simulink model "DUC_SIM"  (R2017b)
settings: Solver=VariableStepAuto  StartTime=0.0  StopTime=10.0  RelTol=1e-3
values from neighbouring files (symbols this model uses):
  A = 0.5*(nLev-1)    (= 0.5)    [Model3.m]
  ftest = 9e3    (= 9000)    [Model3.m]    (also in Model3_LTE.m = 2250)
undefined symbols (not defined in the file or in its folder): a, b, c, g
libraries: dspsigops x16, simulink x8, dspsrcs4 x1
(part 3 of 3)

== matlab function DUC_SIM/Delta_Sigma_Modulator1/Fourth_Order_Delta_Sigma_Modulator_Simulation/MATLAB Function ==
  data: u input; y output
function y = fcn(u)
%#codegen
% nLev=64;
% st=fi(nLev-2,1,36,28);
% y=fi(1,1,36,28);
% for n=1:nLev-2
%     k=fi(n,1,36,28);
%     if u < -st
%         y=fi(-nLev+1,1,36,28);
%         break;
%     elseif u > st
%         y=fi(nLev-1,1,36,28);
%         break;
%     elseif u >= -nLev + 2*k && u <= -nLev + 2*(k+1)
%         y=fi(2*k-1-nLev,1,36,28);
%         break;
%     end
% end

% 2-level
if u < 0
    y = fi(-1,1,36,32);
    %y = -1;
else
    y = fi(1,1,36,32);
    %y = 1;
end

% 4-level
% if u < -2
%     y = fi(-3,1,36,28);
% elseif u > -2 && u < 0
%     y = fi(-1,1,36,28);
% elseif u >= 0 && u < 2
%     y = fi(1,1,36,28);
% else
%     y = fi(3,1,36,28);
% end

% 64-level
% if u < -62
%     y = fi(-63,1,36,28);
% elseif u >= -62 && u < -60
%     y = fi(-61,1,36,28);
% elseif u >= -60 && u < -58
%     y = fi(-59,1,36,28);
% elseif u >= -58 && u < -56
%     y = fi(-57,1,36,28);
% elseif u >= -56 && u < -54
%     y = fi(-55,1,36,28);
% elseif u >= -54 && u < -52
%     y = fi(-53,1,36,28);
% elseif u >= -52 && u < -50
%     y = fi(-51,1,36,28);
% elseif u >= -50 && u < -48
%     y = fi(-49,1,36,28);
% elseif u >= -48 && u < -46
%     y = fi(-47,1,36,28);
% elseif u >= -46 && u < -44
%     y = fi(-45,1,36,28);
% elseif u >= -44 && u < -42
%     y = fi(-43,1,36,28);
% elseif u >= -42 && u < -40
%     y = fi(-41,1,36,28);
% elseif u >= -40 && u < -38
%     y = fi(-39,1,36,28);
% elseif u >= -38 && u < -36
%     y = fi(-37,1,36,28);
% elseif u >= -36 && u < -34
%     y = fi(-35,1,36,28);
% elseif u >= -34 && u < -32
%     y = fi(-33,1,36,28);
% elseif u >= -32 && u < -30
%     y = fi(-31,1,36,28);
% elseif u >= -30 && u < -28
%     y = fi(-29,1,36,28);
% elseif u >= -28 && u < -26
%     y = fi(-27,1,36,28);
% elseif u >= -26 && u < -24
%     y = fi(-25,1,36,28);
% elseif u >= -24 && u < -22
%     y = fi(-23,1,36,28);
% elseif u >= -22 && u < -20
%     y = fi(-21,1,36,28);
% elseif u >= -20 && u < -18
%     y = fi(-19,1,36,28);
% elseif u >= -18 && u < -16
%     y = fi(-17,1,36,28);
% elseif u >= -16 && u < -14
%     y = fi(-15,1,36,28);
% elseif u >= -14 && u < -12
%     y = fi(-13,1,36,28);
% elseif u >= -12 && u < -10
%     y = fi(-11,1,36,28);
% elseif u >= -10 && u < -8
%     y = fi(-9,1,36,28);
% elseif u >= -8 && u < -6
%     y = fi(-7,1,36,28);
% elseif u >= -6 && u < -4
%     y = fi(-5,1,36,28);
% elseif u >= -4 && u < -2
%     y = fi(-3,1,36,28);
% elseif u >= -2 && u < 0
%     y = fi(-1,1,36,28);
% elseif u >= 0 && u < 2
%     y = fi(1,1,36,28);
% elseif u >= 2 && u < 4
%     y = fi(3,1,36,28);
% elseif u >= 4 && u < 6
%     y = fi(5,1,36,28);
% elseif u >= 6 && u < 8
%     y = fi(7,1,36,28);
% elseif u >= 8 && u < 10
%     y = fi(9,1,36,28);
% elseif u >= 10 && u < 12
%     y = fi(11,1,36,28);
% elseif u >= 12 && u < 14
%     y = fi(13,1,36,28);
% elseif u >= 14 && u < 16
%     y = fi(15,1,36,28);
% elseif u >= 16 && u < 18
%     y = fi(17,1,36,28);
% elseif u >= 18 && u < 20
%     y = fi(19,1,36,28);
% elseif u >= 20 && u < 22
%     y = fi(21,1,36,28);
% elseif u >= 22 && u < 24
%     y = fi(23,1,36,28);
% elseif u >= 24 && u < 26
%     y = fi(25,1,36,28);
% elseif u >= 26 && u < 28
%     y = fi(27,1,36,28);
% elseif u >= 28 && u < 30
%     y = fi(29,1,36,28);
% elseif u >= 30 && u < 32
%     y = fi(31,1,36,28);
% elseif u >= 32 && u < 34
%     y = fi(33,1,36,28);
% elseif u >= 34 && u < 36
%     y = fi(35,1,36,28);
% elseif u >= 36 && u < 38
%     y = fi(37,1,36,28);
% elseif u >= 38 && u < 40
%     y = fi(39,1,36,28);
% elseif u >= 40 && u < 42
%     y = fi(41,1,36,28);
% elseif u >= 42 && u < 44
%     y = fi(43,1,36,28);
% elseif u >= 44 && u < 46
%     y = fi(45,1,36,28);
% elseif u >= 46 && u < 48
%     y = fi(47,1,36,28);
% elseif u >= 48 && u < 50
%     y = fi(49,1,36,28);
% elseif u >= 50 && u < 52
%     y = fi(51,1,36,28);
% elseif u >= 52 && u < 54
%     y = fi(53,1,36,28);
% elseif u >= 54 && u < 56
%     y = fi(55,1,36,28);
% elseif u >= 56 && u < 58
%     y = fi(57,1,36,28);
% elseif u >= 58 && u < 60
%     y = fi(59,1,36,28);
% elseif u >= 60 && u < 62
%     y = fi(61,1,36,28);
% else % u > 62
%     y = fi(63,1,36,28);
% end

% 32-level
% if u < -30
%     y = fi(-31,1,36,28);
% elseif u >= -30 && u < -28
%     y = fi(-29,1,36,28);
% elseif u >= -28 && u < -26
%     y = fi(-27,1,36,28);
% elseif u >= -26 && u < -24
%     y = fi(-25,1,36,28);
% elseif u >= -24 && u < -22
%     y = fi(-23,1,36,28);
% elseif u >= -22 && u < -20
%     y = fi(-21,1,36,28);
% elseif u >= -20 && u < -18
%     y = fi(-19,1,36,28);
% elseif u >= -18 && u < -16
%     y = fi(-17,1,36,28);
% elseif u >= -16 && u < -14
%     y = fi(-15,1,36,28);
% elseif u >= -14 && u < -12
%     y = fi(-13,1,36,28);
% elseif u >= -12 && u < -10
%     y = fi(-11,1,36,28);
% elseif u >= -10 && u < -8
%     y = fi(-9,1,36,28);
% elseif u >= -8 && u < -6
%     y = fi(-7,1,36,28);
% elseif u >= -6 && u < -4
%     y = fi(-5,1,36,28);
% elseif u >= -4 && u < -2
%     y = fi(-3,1,36,28);
% elseif u >= -2 && u < 0
%     y = fi(-1,1,36,28);
% elseif u >= 0 && u < 2
%     y = fi(1,1,36,28);
% elseif u >= 2 && u < 4
%     y = fi(3,1,36,28);
% elseif u >= 4 && u < 6
%     y = fi(5,1,36,28);
% elseif u >= 6 && u < 8
%     y = fi(7,1,36,28);
% elseif u >= 8 && u < 10
%     y = fi(9,1,36,28);
% elseif u >= 10 && u < 12
%     y = fi(11,1,36,28);
% elseif u >= 12 && u < 14
%     y = fi(13,1,36,28);
% elseif u >= 14 && u < 16
%     y = fi(15,1,36,28);
% elseif u >= 16 && u < 18
%     y = fi(17,1,36,28);
% elseif u >= 18 && u < 20
%     y = fi(19,1,36,28);
% elseif u >= 20 && u < 22
%     y = fi(21,1,36,28);
% elseif u >= 22 && u < 24
%     y = fi(23,1,36,28);
% elseif u >= 24 && u < 26
%     y = fi(25,1,36,28);
% elseif u >= 26 && u < 28
%     y = fi(27,1,36,28);
% elseif u >= 28 && u < 30
%     y = fi(29,1,36,28);
% else % u > 30
%     y = fi(31,1,36,28);
% end

== matlab function DUC_SIM/Delta_Sigma_Modulator1/Second_Order_Delta_Sigma_Modulator_Simulation/MATLAB Function ==
  data: u input; y output
function y = fcn(u)
%#codegen
% nLev=2;
% st=fi(nLev-2,1,36,30);
% y=fi(0,1,36,30);
% if u < -st
%     y = fi(-nLev+1,1,36,30);
% elseif u >= st
%     y = fi(nLev-1,1,36,30);
% else
%     for n=1:nLev-2
%         k=fi(n,1,36,30);
%         if u >= -nLev + 2*k && u < -nLev + 2*(k+1)
%             y = fi(2*k-1-nLev,1,36,30);
%         end
%     end
% end
% nLev=64;
% st=fi(nLev-2,1,36,25);
% y=fi(0,1,36,25);
% for n=1:nLev-2
%     k=fi(n,1,36,25);
%     if u < -st
%         y = fi(-nLev+1,1,36,25);
%         break;
%     elseif u >= st
%         y = fi(nLev-1,1,36,25);
%         break;
%     elseif u >= -nLev + 2*k && u < -nLev + 2*(k+1)
%         y = fi(2*k-1-nLev,1,36,25);
%         break;
%     end
% end

if u < 0
    y = fi(-1,1,36,32);
    %y = -1;
else
    y = fi(1,1,36,32);
    %y = 1;
end

% if u < -14
%     y = fi(-15,1,36,28);
% elseif u >= -14 && u < -12
%     y = fi(-13,1,36,28);
% elseif u >= -12 && u < -10
%     y = fi(-11,1,36,28);
% elseif u >= -10 && u < -8
%     y = fi(-9,1,36,28);
% elseif u >= -8 && u < -6
%     y = fi(-7,1,36,28);
% elseif u >= -6 && u < -4
%     y = fi(-5,1,36,28);
% elseif u >= -4 && u < -2
%     y = fi(-3,1,36,28);
% elseif u >= -2 && u < 0
%     y = fi(-1,1,36,28);
% elseif u >= 0 && u < 2
%     y = fi(1,1,36,28);
% elseif u >= 2 && u < 4
%     y = fi(3,1,36,28);
% elseif u >= 4 && u < 6
%     y = fi(5,1,36,28);
% elseif u >= 6 && u < 8
%     y = fi(7,1,36,28);
% elseif u >= 8 && u < 10
%     y = fi(9,1,36,28);
% elseif u >= 10 && u < 12
%     y = fi(11,1,36,28);
% elseif u >= 12 && u < 14
%     y = fi(13,1,36,28);
% else % u > 14
%     y = fi(15,1,36,28);
% end

== matlab function DUC_SIM/Delta_Sigma_Modulator2/Eight_Order_Delta_Sigma_Modulator/MATLAB Function ==
  data: u input; y output
function y = fcn(u)
%#codegen
% nLev=32;
% st=fi(nLev-2,1,36,28);
% y=fi(1,1,36,28);
% for n=1:nLev-2
%     k=fi(n,1,36,28);
%     if u < -st
%         y=fi(-nLev+1,1,36,28);
%         break;
%     elseif u > st
%         y=fi(nLev-1,1,36,28);
%         break;
%     elseif u >= -nLev + 2*k && u <= -nLev + 2*(k+1)
%         y=fi(2*k-1-nLev,1,36,28);
%         break;
%     end
% end
% nLev=2;
% st=fi(nLev,1,36,28);
% y=fi(0,1,36,28);
% for n=1:nLev
%     k=fi(n,1,36,28);
%     if u < -st+2
%         y = fi(-nLev+1,1,36,28);
%         break;
%     elseif u < -nLev + 2*k && u > -nLev + 2*(k+1)
%         y = fi(-nLev+1,1,36,28);
%         break;
%     elseif u >= nLev - 2*k && u < nLev - 2*(k+1)
%         y = fi(-nLev+1,1,36,28);
%         break;
%     else u > st-2
%         y = fi(nLev-1,1,36,28);
%         break;
%     end
% end

% 2-level
% if u < 0
%     y = -1;
% else
%     y = 1;
% end

% 2-level
if u < 0
    y = fi(-1,1,36,32);
else
    y = fi(1,1,36,32);
end

% 4-level
% if u < -2
%     y = fi(-3,1,36,28);
% elseif u > -2 && u < 0
%     y = fi(-1,1,36,28);
% elseif u >= 0 && u < 2
%     y = fi(1,1,36,28);
% else
%     y = fi(3,1,36,28);
% end

% 64-level
% if u < -62
%     y = fi(-63,1,36,28);
% elseif u >= -62 && u < -60
%     y = fi(-61,1,36,28);
% elseif u >= -60 && u < -58
%     y = fi(-59,1,36,28);
% elseif u >= -58 && u < -56
%     y = fi(-57,1,36,28);
% elseif u >= -56 && u < -54
%     y = fi(-55,1,36,28);
% elseif u >= -54 && u < -52
%     y = fi(-53,1,36,28);
% elseif u >= -52 && u < -50
%     y = fi(-51,1,36,28);
% elseif u >= -50 && u < -48
%     y = fi(-49,1,36,28);
% elseif u >= -48 && u < -46
%     y = fi(-47,1,36,28);
% elseif u >= -46 && u < -44
%     y = fi(-45,1,36,28);
% elseif u >= -44 && u < -42
%     y = fi(-43,1,36,28);
% elseif u >= -42 && u < -40
%     y = fi(-41,1,36,28);
% elseif u >= -40 && u < -38
%     y = fi(-39,1,36,28);
% elseif u >= -38 && u < -36
%     y = fi(-37,1,36,28);
% elseif u >= -36 && u < -34
%     y = fi(-35,1,36,28);
% elseif u >= -34 && u < -32
%     y = fi(-33,1,36,28);
% elseif u >= -32 && u < -30
%     y = fi(-31,1,36,28);
% elseif u >= -30 && u < -28
%     y = fi(-29,1,36,28);
% elseif u >= -28 && u < -26
%     y = fi(-27,1,36,28);
% elseif u >= -26 && u < -24
%     y = fi(-25,1,36,28);
% elseif u >= -24 && u < -22
%     y = fi(-23,1,36,28);
% elseif u >= -22 && u < -20
%     y = fi(-21,1,36,28);
% elseif u >= -20 && u < -18
%     y = fi(-19,1,36,28);
% elseif u >= -18 && u < -16
%     y = fi(-17,1,36,28);
% elseif u >= -16 && u < -14
%     y = fi(-15,1,36,28);
% elseif u >= -14 && u < -12
%     y = fi(-13,1,36,28);
% elseif u >= -12 && u < -10
%     y = fi(-11,1,36,28);
% elseif u >= -10 && u < -8
%     y = fi(-9,1,36,28);
% elseif u >= -8 && u < -6
%     y = fi(-7,1,36,28);
% elseif u >= -6 && u < -4
%     y = fi(-5,1,36,28);
% elseif u >= -4 && u < -2
%     y = fi(-3,1,36,28);
% elseif u >= -2 && u < 0
%     y = fi(-1,1,36,28);
% elseif u >= 0 && u < 2
%     y = fi(1,1,36,28);
% elseif u >= 2 && u < 4
%     y = fi(3,1,36,28);
% elseif u >= 4 && u < 6
%     y = fi(5,1,36,28);
% elseif u >= 6 && u < 8
%     y = fi(7,1,36,28);
% elseif u >= 8 && u < 10
%     y = fi(9,1,36,28);
% elseif u >= 10 && u < 12
%     y = fi(11,1,36,28);
% elseif u >= 12 && u < 14
%     y = fi(13,1,36,28);
% elseif u >= 14 && u < 16
%     y = fi(15,1,36,28);
% elseif u >= 16 && u < 18
%     y = fi(17,1,36,28);
% elseif u >= 18 && u < 20
%     y = fi(19,1,36,28);
% elseif u >= 20 && u < 22
%     y = fi(21,1,36,28);
% elseif u >= 22 && u < 24
%     y = fi(23,1,36,28);
% elseif u >= 24 && u < 26
%     y = fi(25,1,36,28);
% elseif u >= 26 && u < 28
%     y = fi(27,1,36,28);
% elseif u >= 28 && u < 30
%     y = fi(29,1,36,28);
% elseif u >= 30 && u < 32
%     y = fi(31,1,36,28);
% elseif u >= 32 && u < 34
%     y = fi(33,1,36,28);
% elseif u >= 34 && u < 36
%     y = fi(35,1,36,28);
% elseif u >= 36 && u < 38
%     y = fi(37,1,36,28);
% elseif u >= 38 && u < 40
%     y = fi(39,1,36,28);
% elseif u >= 40 && u < 42
%     y = fi(41,1,36,28);
% elseif u >= 42 && u < 44
%     y = fi(43,1,36,28);
% elseif u >= 44 && u < 46
%     y = fi(45,1,36,28);
% elseif u >= 46 && u < 48
%     y = fi(47,1,36,28);
% elseif u >= 48 && u < 50
%     y = fi(49,1,36,28);
% elseif u >= 50 && u < 52
%     y = fi(51,1,36,28);
% elseif u >= 52 && u < 54
%     y = fi(53,1,36,28);
% elseif u >= 54 && u < 56
%     y = fi(55,1,36,28);
% elseif u >= 56 && u < 58
%     y = fi(57,1,36,28);
% elseif u >= 58 && u < 60
%     y = fi(59,1,36,28);
% elseif u >= 60 && u < 62
%     y = fi(61,1,36,28);
% else % u > 62
%     y = fi(63,1,36,28);
% end

% 32-level
% if u < -30
%     y = fi(-31,1,36,28);
% elseif u >= -30 && u < -28
%     y = fi(-29,1,36,28);
% elseif u >= -28 && u < -26
%     y = fi(-27,1,36,28);
% elseif u >= -26 && u < -24
%     y = fi(-25,1,36,28);
% elseif u >= -24 && u < -22
%     y = fi(-23,1,36,28);
% elseif u >= -22 && u < -20
%     y = fi(-21,1,36,28);
% elseif u >= -20 && u < -18
%     y = fi(-19,1,36,28);
% elseif u >= -18 && u < -16
%     y = fi(-17,1,36,28);
% elseif u >= -16 && u < -14
%     y = fi(-15,1,36,28);
% elseif u >= -14 && u < -12
%     y = fi(-13,1,36,28);
% elseif u >= -12 && u < -10
%     y = fi(-11,1,36,28);
% elseif u >= -10 && u < -8
%     y = fi(-9,1,36,28);
% elseif u >= -8 && u < -6
%     y = fi(-7,1,36,28);
% elseif u >= -6 && u < -4
%     y = fi(-5,1,36,28);
% elseif u >= -4 && u < -2
%     y = fi(-3,1,36,28);
% elseif u >= -2 && u < 0
%     y = fi(-1,1,36,28);
% elseif u >= 0 && u < 2
%     y = fi(1,1,36,28);
% elseif u >= 2 && u < 4
%     y = fi(3,1,36,28);
% elseif u >= 4 && u < 6
%     y = fi(5,1,36,28);
% elseif u >= 6 && u < 8
%     y = fi(7,1,36,28);
% elseif u >= 8 && u < 10
%     y = fi(9,1,36,28);
% elseif u >= 10 && u < 12
%     y = fi(11,1,36,28);
% elseif u >= 12 && u < 14
%     y = fi(13,1,36,28);
% elseif u >= 14 && u < 16
%     y = fi(15,1,36,28);
% elseif u >= 16 && u < 18
%     y = fi(17,1,36,28);
% elseif u >= 18 && u < 20
%     y = fi(19,1,36,28);
% elseif u >= 20 && u < 22
%     y = fi(21,1,36,28);
% elseif u >= 22 && u < 24
%     y = fi(23,1,36,28);
% elseif u >= 24 && u < 26
%     y = fi(25,1,36,28);
% elseif u >= 26 && u < 28
%     y = fi(27,1,36,28);
% elseif u >= 28 && u < 30
%     y = fi(29,1,36,28);
% else % u > 30
%     y = fi(31,1,36,28);
% end

== matlab function DUC_SIM/Delta_Sigma_Modulator2/Fourth_Order_Delta_Sigma_Modulator_Simulation/MATLAB Function ==
  data: u input; y output
function y = fcn(u)
%#codegen
% nLev=64;
% st=fi(nLev-2,1,36,28);
% y=fi(1,1,36,28);
% for n=1:nLev-2
%     k=fi(n,1,36,28);
%     if u < -st
%         y=fi(-nLev+1,1,36,28);
%         break;
%     elseif u > st
%         y=fi(nLev-1,1,36,28);
%         break;
%     elseif u >= -nLev + 2*k && u <= -nLev + 2*(k+1)
%         y=fi(2*k-1-nLev,1,36,28);
%         break;
%     end
% end

% 2-level
if u < 0
    y = fi(-1,1,36,32);
    %y = -1;
else
    y = fi(1,1,36,32);
    %y = 1;
end

% 4-level
% if u < -2
%     y = fi(-3,1,36,28);
% elseif u > -2 && u < 0
%     y = fi(-1,1,36,28);
% elseif u >= 0 && u < 2
%     y = fi(1,1,36,28);
% else
%     y = fi(3,1,36,28);
% end

% 64-level
% if u < -62
%     y = fi(-63,1,36,28);
% elseif u >= -62 && u < -60
%     y = fi(-61,1,36,28);
% elseif u >= -60 && u < -58
%     y = fi(-59,1,36,28);
% elseif u >= -58 && u < -56
%     y = fi(-57,1,36,28);
% elseif u >= -56 && u < -54
%     y = fi(-55,1,36,28);
% elseif u >= -54 && u < -52
%     y = fi(-53,1,36,28);
% elseif u >= -52 && u < -50
%     y = fi(-51,1,36,28);
% elseif u >= -50 && u < -48
%     y = fi(-49,1,36,28);
% elseif u >= -48 && u < -46
%     y = fi(-47,1,36,28);
% elseif u >= -46 && u < -44
%     y = fi(-45,1,36,28);
% elseif u >= -44 && u < -42
%     y = fi(-43,1,36,28);
% elseif u >= -42 && u < -40
%     y = fi(-41,1,36,28);
% elseif u >= -40 && u < -38
%     y = fi(-39,1,36,28);
% elseif u >= -38 && u < -36
%     y = fi(-37,1,36,28);
% elseif u >= -36 && u < -34
%     y = fi(-35,1,36,28);
% elseif u >= -34 && u < -32
%     y = fi(-33,1,36,28);
% elseif u >= -32 && u < -30
%     y = fi(-31,1,36,28);
% elseif u >= -30 && u < -28
%     y = fi(-29,1,36,28);
% elseif u >= -28 && u < -26
%     y = fi(-27,1,36,28);
% elseif u >= -26 && u < -24
%     y = fi(-25,1,36,28);
% elseif u >= -24 && u < -22
%     y = fi(-23,1,36,28);
% elseif u >= -22 && u < -20
%     y = fi(-21,1,36,28);
% elseif u >= -20 && u < -18
%     y = fi(-19,1,36,28);
% elseif u >= -18 && u < -16
%     y = fi(-17,1,36,28);
% elseif u >= -16 && u < -14
%     y = fi(-15,1,36,28);
% elseif u >= -14 && u < -12
%     y = fi(-13,1,36,28);
% elseif u >= -12 && u < -10
%     y = fi(-11,1,36,28);
% elseif u >= -10 && u < -8
%     y = fi(-9,1,36,28);
% elseif u >= -8 && u < -6
%     y = fi(-7,1,36,28);
% elseif u >= -6 && u < -4
%     y = fi(-5,1,36,28);
% elseif u >= -4 && u < -2
%     y = fi(-3,1,36,28);
% elseif u >= -2 && u < 0
%     y = fi(-1,1,36,28);
% elseif u >= 0 && u < 2
%     y = fi(1,1,36,28);
% elseif u >= 2 && u < 4
%     y = fi(3,1,36,28);
% elseif u >= 4 && u < 6
%     y = fi(5,1,36,28);
% elseif u >= 6 && u < 8
%     y = fi(7,1,36,28);
% elseif u >= 8 && u < 10
%     y = fi(9,1,36,28);
% elseif u >= 10 && u < 12
%     y = fi(11,1,36,28);
% elseif u >= 12 && u < 14
%     y = fi(13,1,36,28);
% elseif u >= 14 && u < 16
%     y = fi(15,1,36,28);
% elseif u >= 16 && u < 18
%     y = fi(17,1,36,28);
% elseif u >= 18 && u < 20
%     y = fi(19,1,36,28);
% elseif u >= 20 && u < 22
%     y = fi(21,1,36,28);
% elseif u >= 22 && u < 24
%     y = fi(23,1,36,28);
% elseif u >= 24 && u < 26
%     y = fi(25,1,36,28);
% elseif u >= 26 && u < 28
%     y = fi(27,1,36,28);
% elseif u >= 28 && u < 30
%     y = fi(29,1,36,28);
% elseif u >= 30 && u < 32
%     y = fi(31,1,36,28);
% elseif u >= 32 && u < 34
%     y = fi(33,1,36,28);
% elseif u >= 34 && u < 36
%     y = fi(35,1,36,28);
% elseif u >= 36 && u < 38
%     y = fi(37,1,36,28);
% elseif u >= 38 && u < 40
%     y = fi(39,1,36,28);
% elseif u >= 40 && u < 42
%     y = fi(41,1,36,28);
% elseif u >= 42 && u < 44
%     y = fi(43,1,36,28);
% elseif u >= 44 && u < 46
%     y = fi(45,1,36,28);
% elseif u >= 46 && u < 48
%     y = fi(47,1,36,28);
% elseif u >= 48 && u < 50
%     y = fi(49,1,36,28);
% elseif u >= 50 && u < 52
%     y = fi(51,1,36,28);
% elseif u >= 52 && u < 54
%     y = fi(53,1,36,28);
% elseif u >= 54 && u < 56
%     y = fi(55,1,36,28);
% elseif u >= 56 && u < 58
%     y = fi(57,1,36,28);
% elseif u >= 58 && u < 60
%     y = fi(59,1,36,28);
% elseif u >= 60 && u < 62
%     y = fi(61,1,36,28);
% else % u > 62
%     y = fi(63,1,36,28);
% end

% 32-level
% if u < -30
%     y = fi(-31,1,36,28);
% elseif u >= -30 && u < -28
%     y = fi(-29,1,36,28);
% elseif u >= -28 && u < -26
%     y = fi(-27,1,36,28);
% elseif u >= -26 && u < -24
%     y = fi(-25,1,36,28);
% elseif u >= -24 && u < -22
%     y = fi(-23,1,36,28);
% elseif u >= -22 && u < -20
%     y = fi(-21,1,36,28);
% elseif u >= -20 && u < -18
%     y = fi(-19,1,36,28);
% elseif u >= -18 && u < -16
%     y = fi(-17,1,36,28);
% elseif u >= -16 && u < -14
%     y = fi(-15,1,36,28);
% elseif u >= -14 && u < -12
%     y = fi(-13,1,36,28);
% elseif u >= -12 && u < -10
%     y = fi(-11,1,36,28);
% elseif u >= -10 && u < -8
%     y = fi(-9,1,36,28);
% elseif u >= -8 && u < -6
%     y = fi(-7,1,36,28);
% elseif u >= -6 && u < -4
%     y = fi(-5,1,36,28);
% elseif u >= -4 && u < -2
%     y = fi(-3,1,36,28);
% elseif u >= -2 && u < 0
%     y = fi(-1,1,36,28);
% elseif u >= 0 && u < 2
%     y = fi(1,1,36,28);
% elseif u >= 2 && u < 4
%     y = fi(3,1,36,28);
% elseif u >= 4 && u < 6
%     y = fi(5,1,36,28);
% elseif u >= 6 && u < 8
%     y = fi(7,1,36,28);
% elseif u >= 8 && u < 10
%     y = fi(9,1,36,28);
% elseif u >= 10 && u < 12
%     y = fi(11,1,36,28);
% elseif u >= 12 && u < 14
%     y = fi(13,1,36,28);
% elseif u >= 14 && u < 16
%     y = fi(15,1,36,28);
% elseif u >= 16 && u < 18
%     y = fi(17,1,36,28);
% elseif u >= 18 && u < 20
%     y = fi(19,1,36,28);
% elseif u >= 20 && u < 22
%     y = fi(21,1,36,28);
% elseif u >= 22 && u < 24
%     y = fi(23,1,36,28);
% elseif u >= 24 && u < 26
%     y = fi(25,1,36,28);
% elseif u >= 26 && u < 28
%     y = fi(27,1,36,28);
% elseif u >= 28 && u < 30
%     y = fi(29,1,36,28);
% else % u > 30
%     y = fi(31,1,36,28);
% end

== matlab function DUC_SIM/Delta_Sigma_Modulator2/Second_Order_Delta_Sigma_Modulator_Simulation/MATLAB Function ==
  data: u input; y output
function y = fcn(u)
%#codegen
% nLev=2;
% st=fi(nLev-2,1,36,30);
% y=fi(0,1,36,30);
% if u < -st
%     y = fi(-nLev+1,1,36,30);
% elseif u >= st
%     y = fi(nLev-1,1,36,30);
% else
%     for n=1:nLev-2
%         k=fi(n,1,36,30);
%         if u >= -nLev + 2*k && u < -nLev + 2*(k+1)
%             y = fi(2*k-1-nLev,1,36,30);
%         end
%     end
% end
% nLev=64;
% st=fi(nLev-2,1,36,25);
% y=fi(0,1,36,25);
% for n=1:nLev-2
%     k=fi(n,1,36,25);
%     if u < -st
%         y = fi(-nLev+1,1,36,25);
%         break;
%     elseif u >= st
%         y = fi(nLev-1,1,36,25);
%         break;
%     elseif u >= -nLev + 2*k && u < -nLev + 2*(k+1)
%         y = fi(2*k-1-nLev,1,36,25);
%         break;
%     end
% end

if u < 0
    y = fi(-1,1,36,32);
    %y = -1;
else
    y = fi(1,1,36,32);
    %y = 1;
end

% if u < -14
%     y = fi(-15,1,36,28);
% elseif u >= -14 && u < -12
%     y = fi(-13,1,36,28);
% elseif u >= -12 && u < -10
%     y = fi(-11,1,36,28);
% elseif u >= -10 && u < -8
%     y = fi(-9,1,36,28);
% elseif u >= -8 && u < -6
%     y = fi(-7,1,36,28);
% elseif u >= -6 && u < -4
%     y = fi(-5,1,36,28);
% elseif u >= -4 && u < -2
%     y = fi(-3,1,36,28);
% elseif u >= -2 && u < 0
%     y = fi(-1,1,36,28);
% elseif u >= 0 && u < 2
%     y = fi(1,1,36,28);
% elseif u >= 2 && u < 4
%     y = fi(3,1,36,28);
% elseif u >= 4 && u < 6
%     y = fi(5,1,36,28);
% elseif u >= 6 && u < 8
%     y = fi(7,1,36,28);
% elseif u >= 8 && u < 10
%     y = fi(9,1,36,28);
% elseif u >= 10 && u < 12
%     y = fi(11,1,36,28);
% elseif u >= 12 && u < 14
%     y = fi(13,1,36,28);
% else % u > 14
%     y = fi(15,1,36,28);
% end
